simulink model "LinearDiscreteStateSpaceModelLQR"  (R2014b)
settings: Solver=ode45  StartTime=0.0  StopTime=100  RelTol=1e-6
undefined symbols (not defined in the file): discrete_state_space_model, lqr_gain_discrete
settings Model: Creator=NagyZe  LastModifiedBy=levente.nagy960115

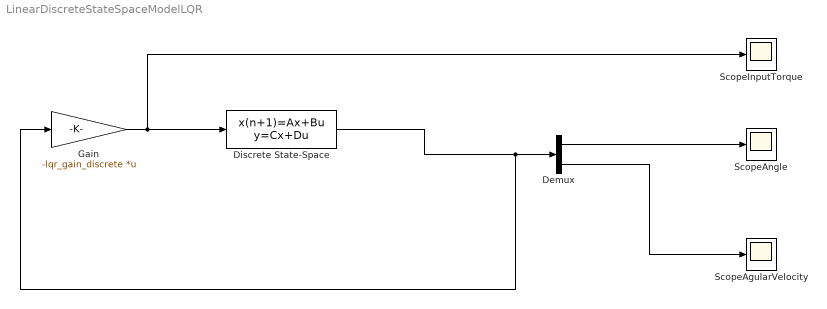
== system LinearDiscreteStateSpaceModelLQR ==
  Demux : Demux  Outputs=2
  Discrete State-Space : DiscreteStateSpace  A=discrete_state_space_model.A  B=discrete_state_space_model.B  C=eye(4)  D=zeros(4,2)  X0=[0.2 0.3 0 0]
  Gain : Gain  Gain=-lqr_gain_discrete  Multiplication=Matrix(K*u) (u vector)
  ScopeAgularVelocity : Scope
      settings: TimeRange=10  YMin=-40  YMax=30  SaveName=jointVelocity
  ScopeAngle : Scope
      settings: TimeRange=10  YMin=-0.005  YMax=0.03  SaveName=jointAngle
  ScopeInputTorque : Scope
      settings: YMin=-1  YMax=1  SaveName=torque
  wires:
  Gain/1 -> Discrete State-Space/1, ScopeInputTorque/1
  Discrete State-Space/1 -> Gain/1, Demux/1
  Demux/1 -> ScopeAngle/1
  Demux/2 -> ScopeAgularVelocity/1
